simulink model "New"
settings: Solver=ode45  SolverMode=SingleTasking  StartTime=0.0  StopTime=1  RelTol=1e-3
values from neighbouring files (symbols this model uses):
  f = 0    [Exercise7.m]
  J = Jtot    (= 2.66691358025e-06)    [Exercise7.m]
  ke = 0.0278    [Exercise7.m]
  kt = 0.0278    [Exercise7.m]
  L = 0    [Exercise7.m]
  N = 45    [Exercise7.m]
  R = 9.73    [Exercise7.m]
libraries: ADDAlib x2
settings Model: Creator=Ramiro  LastModifiedBy=k340h17
settings DataIOCC: LimitDataPoints=on  SaveFormat=Array  SignalLoggingSaveFormat=ModelDataLogs  ReturnWorkspaceOutputs=off
settings OptimizationCC: BlockReduction=off  BooleanDataType=off  ExpressionDepthLimit=2147483647  LifeSpan=inf  SimCompilerOptimization=Off
settings DebuggingCC: SaveWithParameterizedLinksMsg=none  UnderspecifiedInitializationDetection=Classic  MergeDetectMultiDrivingBlocksExec=none  SignalResolutionControl=TryResolveAllWithWarning  MultiTaskDSMMsg=warning  MultiTaskCondExecSysMsg=none  FcnCallInpInsideContextMsg=Enable All  FrameProcessingCompatibilityMsg=warning  StateNameClashWarn=warning  StrictBusMsg=None  SFUnexpectedBacktrackingDiag=warning  SFNoUnconditionalDefaultTransitionDiag=warning
settings HardwareCC: ProdBitPerPointer=32  ProdLargestAtomicFloat=None  ProdIntDivRoundTo=Undefined  ProdEndianess=Unspecified  ProdWordSize=32  ProdHWDeviceType=32-bit Generic  TargetUnknown=on
settings ModelReferenceCC: PropagateSignalLabelsOutOfModel=off
settings SFSimCC: SimUseLocalCustomCode=off
settings RTWCC: RTWUseLocalCustomCode=off  IncludeERTFirstTime=on  RTWCompilerOptimization=Off
settings CodeAppCC: CustomSymbolStrType=$N$R$M
settings GRTTargetCC: CodeReplacementLibrary=ANSI_C  GeneratePreprocessorConditionals=Disable all  CPPClassGenCompliant=off

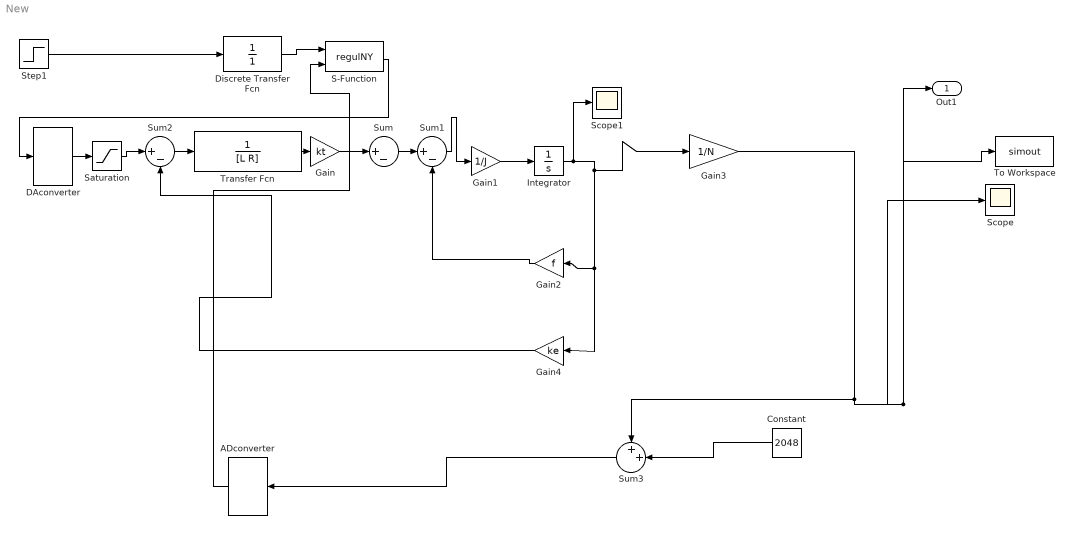
== system New ==
  ADconverter : ADDAlib/ADconverter  Vinmin=-10  Vinmax=9.995  ADoutmin=0  ADoutmax=4095  Tsample=0.01
  Constant : Constant  Value=2048
  DAconverter : ADDAlib/DAconverter  Voutmin=-10  Voutmax=9.995  DAinmin=0  DAinmax=4095  Tsample=.00525
  Discrete Transfer Fcn : DiscreteTransferFcn  Denominator=[1]  SampleTime=.00525
  Gain : Gain  Gain=kt
  Gain1 : Gain  Gain=1/J
  Gain2 : Gain  Gain=f
  Gain3 : Gain  Gain=1/N
  Gain4 : Gain  Gain=ke
  Integrator : Integrator
  S-Function : S-Function  FunctionName=regulNY  Parameters=1.071 -0.9286 -1  EnableBusSupport=off
  Saturation : Saturate  UpperLimit=10  LowerLimit=-10
  Scope : Scope
  Scope1 : Scope
  Step1 : Step  SampleTime=0
  Sum : Sum  Inputs=|+-
  Sum1 : Sum  Inputs=|+-
  Sum2 : Sum  Inputs=|+-
  Sum3 : Sum  Inputs=++|
  To Workspace : ToWorkspace  VariableName=simout  SampleTime=-1  SaveFormat=Structure With Time
  Transfer Fcn : TransferFcn  Denominator=[L R]
  Out1 : Outport
  wires:
  Sum/1 -> Sum1/1
  Sum1/1 -> Gain1/1
  Gain2/1 -> Sum1/2
  Transfer Fcn/1 -> Gain/1
  Sum2/1 -> Transfer Fcn/1
  Gain1/1 -> Integrator/1
  Integrator/1 -> Gain4/1, Gain2/1, Gain3/1, Scope1/1
  Gain3/1 -> Out1/1, Scope/1, To Workspace/1, Sum3/1
  Gain/1 -> Sum/1
  Saturation/1 -> Sum2/1
  Step1/1 -> Discrete Transfer Fcn/1
  DAconverter/1 -> Saturation/1
  S-Function/1 -> DAconverter/1
  Gain4/1 -> Sum2/2
  ADconverter/1 -> S-Function/2
  Discrete Transfer Fcn/1 -> S-Function/1
  Sum3/1 -> ADconverter/1
  Constant/1 -> Sum3/2
